simulink model "beam_control_ic_tx"  (R2022b)
settings: Solver=FixedStepAuto  StartTime=0.0  StopTime=100e-7  RelTol=1e-3
values from neighbouring files (symbols this model uses):
  beam_former_gain_array = [1 1]    [beam_control_ic_tx_parameter.m]
  Bias = 0    [ModelingRFSystemsWithAntennaArraysUsingAntennaBlockExample.m]    (also in beam_control_ic_rx_parameter.m)
  filter_gain0_0 = 0    [ModelingRFSystemsWithAntennaArraysUsingAntennaBlockExample.m]    (also in beam_control_ic_rx_parameter.m)
  filter_gain0_1 = 1/6    (= 0.166666666667)    [ModelingRFSystemsWithAntennaArraysUsingAntennaBlockExample.m]    (also in beam_control_ic_rx_parameter.m)
  filter_gain0_2 = 2/3    (= 0.666666666667)    [ModelingRFSystemsWithAntennaArraysUsingAntennaBlockExample.m]    (also in beam_control_ic_rx_parameter.m)
  filter_gain0_3 = 1/6    (= 0.166666666667)    [ModelingRFSystemsWithAntennaArraysUsingAntennaBlockExample.m]    (also in beam_control_ic_rx_parameter.m)
  filter_gain1_0 = 0    [ModelingRFSystemsWithAntennaArraysUsingAntennaBlockExample.m]    (also in beam_control_ic_rx_parameter.m)
  filter_gain1_1 = 1/2    (= 0.5)    [ModelingRFSystemsWithAntennaArraysUsingAntennaBlockExample.m]    (also in beam_control_ic_rx_parameter.m)
  filter_gain1_2 = 0    [ModelingRFSystemsWithAntennaArraysUsingAntennaBlockExample.m]    (also in beam_control_ic_rx_parameter.m)
  filter_gain1_3 = -1/2    (= -0.5)    [ModelingRFSystemsWithAntennaArraysUsingAntennaBlockExample.m]    (also in beam_control_ic_rx_parameter.m)
  filter_gain2_0 = 0    [ModelingRFSystemsWithAntennaArraysUsingAntennaBlockExample.m]    (also in beam_control_ic_rx_parameter.m)
  filter_gain2_1 = 1/2    (= 0.5)    [ModelingRFSystemsWithAntennaArraysUsingAntennaBlockExample.m]    (also in beam_control_ic_rx_parameter.m)
  filter_gain2_2 = -1    [ModelingRFSystemsWithAntennaArraysUsingAntennaBlockExample.m]    (also in beam_control_ic_rx_parameter.m)
  filter_gain2_3 = 1/2    (= 0.5)    [ModelingRFSystemsWithAntennaArraysUsingAntennaBlockExample.m]    (also in beam_control_ic_rx_parameter.m)
  filter_gain3_0 = 1/6    (= 0.166666666667)    [ModelingRFSystemsWithAntennaArraysUsingAntennaBlockExample.m]    (also in beam_control_ic_rx_parameter.m)
  filter_gain3_1 = -1/2    (= -0.5)    [ModelingRFSystemsWithAntennaArraysUsingAntennaBlockExample.m]    (also in beam_control_ic_rx_parameter.m)
  filter_gain3_2 = 1/2    (= 0.5)    [ModelingRFSystemsWithAntennaArraysUsingAntennaBlockExample.m]    (also in beam_control_ic_rx_parameter.m)
  filter_gain3_3 = -1/6    (= -0.166666666667)    [ModelingRFSystemsWithAntennaArraysUsingAntennaBlockExample.m]    (also in beam_control_ic_rx_parameter.m)
  fraction_delay = 1.5    [ModelingRFSystemsWithAntennaArraysUsingAntennaBlockExample.m]    (also in beam_control_ic_rx_parameter.m = 1)
  integer_delay = 0    [ModelingRFSystemsWithAntennaArraysUsingAntennaBlockExample.m]    (also in beam_control_ic_rx_parameter.m)
  N = 10    [ModelingRFSystemsWithAntennaArraysUsingAntennaBlockExample.m]    (also in beam_control_ic_rx_parameter.m)
  Ref = 2.048    [ModelingRFSystemsWithAntennaArraysUsingAntennaBlockExample.m]    (also in beam_control_ic_rx_parameter.m)
undefined symbols (not defined in the file or in its folder): fdesignblkfcn, gcbh, pskmod
libraries: dspsigops x5, simulink_extras x2, msbDacArchitectures x2, dspmlti4 x2, commrfcorlib x2, commeq3 x2
(part 2 of 2)

== system beam_control_ic_tx/DAC4/Bandpass Filter ==
  In : Inport
  Generated Filter Block : DiscreteFir  Tag=BlockMethodSubSystem  Coefficients=[-0.0012202546535986659 -9.13233975482966975e-05 -8.99256829754742885e-05 -8.49568620794813187e-05 -7.65918257031608733e-05 -6.45471094074974157e-05 -4.91277813323746533e-05 -3.02130898541744078e-05 -8.26870645732298906e-06 1.6671662698626823e-05 4.39541890279793922e-05 7.34165310252373626e-05 0.00010423396503717428 0.000136131752137668013 0.000168143983641900536 0.000199929301866810821 0.000230438299035856507 0.000259337821459698441 0.000285558345357348343 0.000308854056151249348 0.000328191318878406837 0.000343487740105433061 0.000353783444423518966 0.000359216150843886357 0.000358877385931074167 0.000353153894755522967 0.000341097824774017966 0.000323462433785893437 0.000299153561126560717 0.000269745115882802052 0.000233999040919835073 0.0001972004364277001 0.000153515870533658326 0.000106052383174717454 5.74539683352688965e-05 6.04594937650455504e-06 -4.55532310469031223e-05 -9.75908830675224862e-05 -0.000148164093683745521 -0.000197070528565657208 -0.000242728118736851024 -0.000284776264896170034 -0.000321913989092721144 -0.000353815467052420176 -0.000379481351760147412 -0.000398736321258097014 -0.00041090935752302718 -0.000416047689810445103 -0.000413829220850846398 -0.000404555890701169198 -0.000388248269640107876 -0.000365462957470535194 -0.000336548652296022525 -0.000302316329255797496 -0.000263442046145281243 -0.000220963786115195229 -0.000175834314391773748 -0.000129161025471032434 -8.20231350887763982e-05 -3.53296492329255448e-05 9.84302486310524778e-06 5.27589512878009519e-05 9.15832635101325855e-05 0.00012581932856439563 0.000155792459998817305 0.000179311417069102214 0.000197211587926015658 0.000208470437254843892 0.000213601308435843601 0.000212295092470561223 0.000205291834434040416 0.000192778620608964287 0.000175776545636206701 0.000154858426385196885 0.000131308335455560313 0.000105981578865262677 8.03397623547331925e-05 5.53951919944831178e-05 3.26700953607227674e-05 1.32031575697712826e-05 -1.55402099136601001e-06 -1.06909266062913088e-05 -1.29935548850691748e-05 -7.86193617095907061e-06 5.5089222371036099e-06 2.72757854722344067e-05 5.77406106991189529e-05 9.65836890737276771e-05 0.000143559362790120345 0.000197828250645135524 0.000258495593684375611 0.000324010131086399015 0.000392854280153913458 0.000463150727242514428 0.000533418473468094722 0.000600454530368638812 0.000662791384862946339 0.000717520719571266533 0.000762479769721939658 0.000795116068628058214 0.000813337209861430123 0.000814900266159901865 0.000798108096414434009 0.000761260178134740072 0.000703325174504752099 0.000623364666425130416 0.000521218788733225809 0.000396901861082561279 0.000251290140065027544 8.54860242376265418e-05 -9.85186714642339537e-05 -0.000298513730639542283 -0.000511433388823435845 -0.00073404891483466793 -0.000962347845386558724 -0.00119223211821992007 -0.0014189389136464621 -0.00163774257621570186 -0.00184346026418805652 -0.00203113725957193483 -0.00219560372436551372 -0.00233214315770362062 -0.00243586822859980347 -0.00250263356215136646 -0.00252835677828219113 -0.00251033906985934216 -0.00244549307869462718 -0.0023323464687573024 -0.00216991176878318388 -0.00195816325575549378 -0.00169805456052523718 -0.00139156861909342099 -0.00104161585514164984 -0.000652217381061162625 -0.000228229107151013526 0.000224397266708858896 0.000699039314055165378 0.00118811737340007695 0.00168360791214046011 0.00217675318553171978 0.00265862218983287232 0.0031198341925478012 0.00355115786310887136 0.00394325828722860358 0.00428731586402832012 0.00457478741725708508 0.00479799989507451261 0.00494991639529222295 0.00502467947522689407 0.00501739055637637731 0.00492463257395766175 0.00474420566528107549 0.00447571265924948634 0.004119974607956183 0.00367973510975244059 0.00315898227276344666 0.00256385576315171964 0.00190158229186866636 0.00118104038765279762 0.000412596290848017374 -0.000392334238645677751 -0.00122117229085016207 -0.00206045828942050258 -0.00289614333571111505 -0.00371365814433393098 -0.00449839785149659926 ...(+7778 chars)]  InputProcessing=Columns as channels (frame based)
  Out : Outport  VectorParamsAs1DForOutWhenUnconnected=off
  wires:
  Generated Filter Block/1 -> Out/1
  In/1 -> Generated Filter Block/1

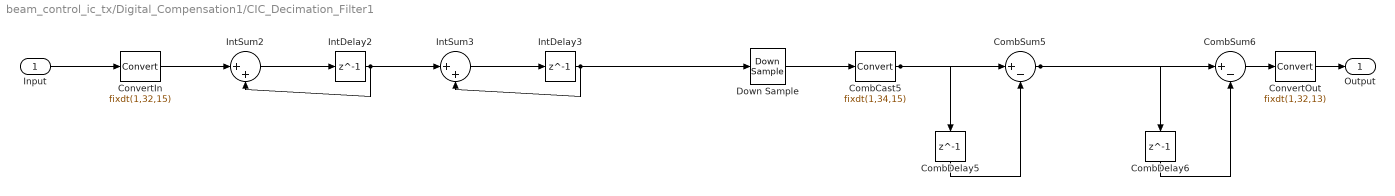
== system beam_control_ic_tx/Digital_Compensation1/CIC_Decimation_Filter1 ==
  Input : Inport
  CombCast5 : DataTypeConversion  OutDataTypeStr=fixdt(1,34,15)  SaturateOnIntegerOverflow=off  RndMeth=Floor
  CombDelay5 : Delay  DelayLength=1  InitialCondition=0
  CombDelay6 : Delay  DelayLength=1  InitialCondition=0
  CombSum5 : Sum  Inputs=|+-  AccumDataTypeStr=fixdt(1,34,15)  OutDataTypeStr=fixdt(1,34,15)
  CombSum6 : Sum  Inputs=|+-  AccumDataTypeStr=fixdt(1,34,15)  OutDataTypeStr=fixdt(1,34,15)
  ConvertIn : DataTypeConversion  OutDataTypeStr=fixdt(1,32,15)  RndMeth=Nearest
  ConvertOut : DataTypeConversion  OutDataTypeStr=fixdt(1,32,13)  SaturateOnIntegerOverflow=off  RndMeth=Floor
  Down Sample : DownSample  RateOptions=Allow multirate processing  AllowArbitraryFixedInput=on
  IntDelay2 : Delay  DelayLength=1  InitialCondition=0
  IntDelay3 : Delay  DelayLength=1  InitialCondition=0
  IntSum2 : Sum  Inputs=|++  AccumDataTypeStr=fixdt(1,34,15)  OutDataTypeStr=fixdt(1,34,15)
  IntSum3 : Sum  Inputs=|++  AccumDataTypeStr=fixdt(1,34,15)  OutDataTypeStr=fixdt(1,34,15)
  Output : Outport
  wires:
  ConvertOut/1 -> Output/1
  CombDelay6/1 -> CombSum6/2
  CombSum6/1 -> ConvertOut/1
  CombCast5/1 -> CombDelay5/1, CombSum5/1
  CombDelay5/1 -> CombSum5/2
  CombSum5/1 -> CombDelay6/1, CombSum6/1
  Down Sample/1 -> CombCast5/1
  IntDelay3/1 -> Down Sample/1, IntSum3/2
  IntSum3/1 -> IntDelay3/1
  IntDelay2/1 -> IntSum3/1, IntSum2/2
  IntSum2/1 -> IntDelay2/1
  ConvertIn/1 -> IntSum2/1
  Input/1 -> ConvertIn/1

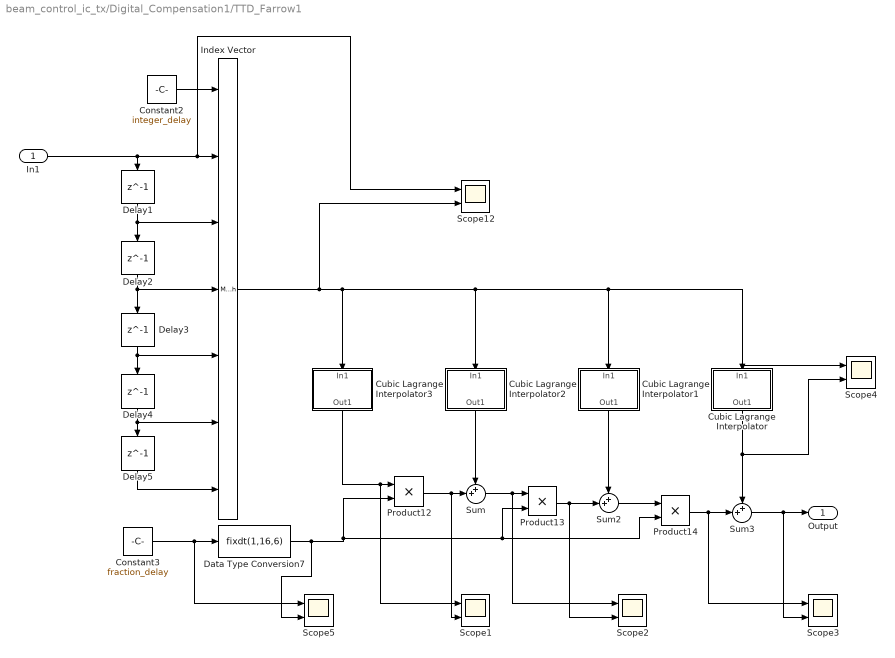
== system beam_control_ic_tx/Digital_Compensation1/TTD_Farrow1 ==
  In1 : Inport
  Constant2 : Constant  Value=integer_delay
  Constant3 : Constant  Value=fraction_delay
  Cubic Lagrange Interpolator : Subsystem
  Cubic Lagrange Interpolator1 : Subsystem
  Cubic Lagrange Interpolator2 : Subsystem
  Cubic Lagrange Interpolator3 : Subsystem
  Data Type Conversion7 : DataTypeConversion  OutDataTypeStr=fixdt(1,16,6)  SaturateOnIntegerOverflow=off  RndMeth=Floor
  Delay{1..5} (5 alike) : Delay  DelayLength=1
  Index Vector : MultiPortSwitch  DataPortOrder=Zero-based contiguous  Inputs=6  zeroidx=on  SaturateOnIntegerOverflow=off  InputSameDT=off
  Product12 : Product
  Product13 : Product
  Product14 : Product
  Scope{1..5,12} (6 alike) : Scope  NumInputPorts=2
  Sum : Sum  Inputs=++|
  Sum2 : Sum  Inputs=++|
  Sum3 : Sum  Inputs=++|
  Output : Outport
  wires:
  Constant3/1 -> Scope5/1, Data Type Conversion7/1
  Cubic Lagrange Interpolator2/1(Out1) -> Sum/1
  Cubic Lagrange Interpolator/1(Out1) -> Scope4/2, Sum3/1
  Sum3/1 -> Scope3/2, Output/1
  In1/1 -> Delay1/1, Scope12/1, Index Vector/2
  Delay2/1 -> Index Vector/4, Delay3/1
  Product13/1 -> Scope2/2, Sum2/2
  Delay1/1 -> Delay2/1, Index Vector/3
  Delay3/1 -> Delay4/1, Index Vector/5
  Delay4/1 -> Delay5/1, Index Vector/6
  Sum2/1 -> Product14/1
  Cubic Lagrange Interpolator3/1(Out1) -> Scope1/1, Product12/1
  Delay5/1 -> Index Vector/7
  Constant2/1 -> Index Vector/1
  Index Vector/1 -> Scope12/2, Scope4/1, Cubic Lagrange Interpolator/1(In1), Cubic Lagrange Interpolator1/1(In1), Cubic Lagrange Interpolator2/1(In1), Cubic Lagrange Interpolator3/1(In1)
  Product12/1 -> Scope1/2, Sum/2
  Cubic Lagrange Interpolator1/1(Out1) -> Sum2/1
  Product14/1 -> Scope3/1, Sum3/2
  Sum/1 -> Scope2/1, Product13/1
  Data Type Conversion7/1 -> Scope5/2, Product14/2, Product13/2, Product12/2

== system beam_control_ic_tx/Digital_Compensation4/CIC_Decimation_Filter3 ==
  Input : Inport
  CombCast5 : DataTypeConversion  OutDataTypeStr=fixdt(1,34,15)  SaturateOnIntegerOverflow=off  RndMeth=Floor
  CombDelay5 : Delay  DelayLength=1  InitialCondition=0
  CombDelay6 : Delay  DelayLength=1  InitialCondition=0
  CombSum5 : Sum  Inputs=|+-  AccumDataTypeStr=fixdt(1,34,15)  OutDataTypeStr=fixdt(1,34,15)
  CombSum6 : Sum  Inputs=|+-  AccumDataTypeStr=fixdt(1,34,15)  OutDataTypeStr=fixdt(1,34,15)
  ConvertIn : DataTypeConversion  OutDataTypeStr=fixdt(1,32,15)  RndMeth=Nearest
  ConvertOut : DataTypeConversion  OutDataTypeStr=fixdt(1,32,13)  SaturateOnIntegerOverflow=off  RndMeth=Floor
  Down Sample : DownSample  RateOptions=Allow multirate processing  AllowArbitraryFixedInput=on
  IntDelay2 : Delay  DelayLength=1  InitialCondition=0
  IntDelay3 : Delay  DelayLength=1  InitialCondition=0
  IntSum2 : Sum  Inputs=|++  AccumDataTypeStr=fixdt(1,34,15)  OutDataTypeStr=fixdt(1,34,15)
  IntSum3 : Sum  Inputs=|++  AccumDataTypeStr=fixdt(1,34,15)  OutDataTypeStr=fixdt(1,34,15)
  Output : Outport
  wires:
  ConvertOut/1 -> Output/1
  CombDelay6/1 -> CombSum6/2
  CombSum6/1 -> ConvertOut/1
  CombCast5/1 -> CombDelay5/1, CombSum5/1
  CombDelay5/1 -> CombSum5/2
  CombSum5/1 -> CombDelay6/1, CombSum6/1
  Down Sample/1 -> CombCast5/1
  IntDelay3/1 -> Down Sample/1, IntSum3/2
  IntSum3/1 -> IntDelay3/1
  IntDelay2/1 -> IntSum3/1, IntSum2/2
  IntSum2/1 -> IntDelay2/1
  ConvertIn/1 -> IntSum2/1
  Input/1 -> ConvertIn/1

== system beam_control_ic_tx/Digital_Compensation1/TTD_Farrow1/Cubic Lagrange Interpolator ==
  In1 : Inport
  Delay6 : Delay  DelayLength=1
  Delay7 : Delay  DelayLength=1
  Delay8 : Delay  DelayLength=1
  Gain : Gain  Gain=filter_gain0_3
  Gain1 : Gain  Gain=filter_gain0_2
  Gain2 : Gain  Gain=filter_gain0_1
  Gain3 : Gain  Gain=filter_gain0_0
  Scope2 : Scope  NumInputPorts=3
  Sum : Sum  Inputs=++|
  Sum2 : Sum  Inputs=++|
  Sum3 : Sum  Inputs=++|
  Out1 : Outport
  wires:
  Sum3/1 -> Scope2/2, Out1/1
  Gain3/1 -> Sum3/1
  Sum/1 -> Sum2/2
  Gain/1 -> Sum/2
  Delay8/1 -> Gain3/1
  In1/1 -> Scope2/3, Delay6/1, Gain/1
  Gain2/1 -> Sum2/1
  Sum2/1 -> Scope2/1, Sum3/2
  Delay7/1 -> Gain2/1, Delay8/1
  Delay6/1 -> Gain1/1, Delay7/1
  Gain1/1 -> Sum/1

== system beam_control_ic_tx/Digital_Compensation1/TTD_Farrow1/Cubic Lagrange Interpolator1 ==
  In1 : Inport
  Delay6 : Delay  DelayLength=1
  Delay7 : Delay  DelayLength=1
  Delay8 : Delay  DelayLength=1
  Gain : Gain  Gain=filter_gain1_3
  Gain1 : Gain  Gain=filter_gain1_2
  Gain2 : Gain  Gain=filter_gain1_1
  Gain3 : Gain  Gain=filter_gain1_0
  Sum : Sum  Inputs=++|
  Sum2 : Sum  Inputs=++|
  Sum3 : Sum  Inputs=++|
  Out1 : Outport
  wires:
  Gain1/1 -> Sum/1
  Delay6/1 -> Delay7/1, Gain1/1
  Delay7/1 -> Delay8/1, Gain2/1
  Sum2/1 -> Sum3/2
  Gain2/1 -> Sum2/1
  In1/1 -> Gain/1, Delay6/1
  Delay8/1 -> Gain3/1
  Gain/1 -> Sum/2
  Sum/1 -> Sum2/2
  Gain3/1 -> Sum3/1
  Sum3/1 -> Out1/1

== system beam_control_ic_tx/Digital_Compensation1/TTD_Farrow1/Cubic Lagrange Interpolator2 ==
  In1 : Inport
  Delay6 : Delay  DelayLength=1
  Delay7 : Delay  DelayLength=1
  Delay8 : Delay  DelayLength=1
  Gain : Gain  Gain=filter_gain2_3
  Gain1 : Gain  Gain=filter_gain2_2
  Gain2 : Gain  Gain=filter_gain2_1
  Gain3 : Gain  Gain=filter_gain2_0
  Sum : Sum  Inputs=++|
  Sum2 : Sum  Inputs=++|
  Sum3 : Sum  Inputs=++|
  Out1 : Outport
  wires:
  Sum3/1 -> Out1/1
  Gain3/1 -> Sum3/1
  Sum/1 -> Sum2/2
  Gain/1 -> Sum/2
  Delay8/1 -> Gain3/1
  In1/1 -> Delay6/1, Gain/1
  Gain2/1 -> Sum2/1
  Sum2/1 -> Sum3/2
  Delay7/1 -> Gain2/1, Delay8/1
  Delay6/1 -> Gain1/1, Delay7/1
  Gain1/1 -> Sum/1

== system beam_control_ic_tx/Digital_Compensation1/TTD_Farrow1/Cubic Lagrange Interpolator3 ==
  In1 : Inport
  Delay6 : Delay  DelayLength=1
  Delay7 : Delay  DelayLength=1
  Delay8 : Delay  DelayLength=1
  Gain : Gain  Gain=filter_gain3_3
  Gain1 : Gain  Gain=filter_gain3_2
  Gain2 : Gain  Gain=filter_gain3_1
  Gain3 : Gain  Gain=filter_gain3_0
  Sum : Sum  Inputs=++|
  Sum2 : Sum  Inputs=++|
  Sum3 : Sum  Inputs=++|
  Out1 : Outport
  wires:
  Gain1/1 -> Sum/1
  Delay6/1 -> Delay7/1, Gain1/1
  Delay7/1 -> Delay8/1, Gain2/1
  Sum2/1 -> Sum3/2
  Gain2/1 -> Sum2/1
  In1/1 -> Gain/1, Delay6/1
  Delay8/1 -> Gain3/1
  Gain/1 -> Sum/2
  Sum/1 -> Sum2/2
  Gain3/1 -> Sum3/1
  Sum3/1 -> Out1/1
